simulink model "reaktor_nastawy"  (R2016a)
settings: Solver=VariableStepAuto  StartTime=0.0  StopTime=500  RelTol=1e-3
values from neighbouring files (symbols this model uses):
  B = 0.0064    [Unit_3.m]    (also in reactor_pocz.m; unit_1.m; unit_4.m)
  C_psi = 13.75 * (10 ^ 6)    (= 13750000)    [Unit_3.m]    (also in reactor_pocz.m; unit_4.m)
  LAMBDA = 10 ^ -5    (= 1e-05)    [Unit_3.m]    (also in reactor_pocz.m; unit_1.m; unit_4.m)
  lambda = 0.1    [Unit_3.m]    (also in reactor_pocz.m; unit_1.m; unit_4.m)
  P_1 = -1.223 * (10 ^ -4)    (= -0.0001223)    [Unit_3.m]    (also in reactor_pocz.m; unit_1.m = -0.0001322; unit_4.m = -0.0001286)
  P_2 = -5.502 * (10 ^ -5)    (= -5.502e-05)    [Unit_3.m]    (also in reactor_pocz.m; unit_1.m = -6.08e-05; unit_4.m = -6.79e-05)
  P_3 = -1.953 * (10 ^ -4)    (= -0.0001953)    [Unit_3.m]    (also in reactor_pocz.m; unit_1.m = -0.000285; unit_4.m = -0.0002887)
  S = 1938.9    [Unit_3.m]    (also in reactor_pocz.m; unit_1.m = 2859; unit_4.m = 2910.3)
libraries: simulink x2
settings Model: Creator=Użytkownik  LastModifiedBy=Użytkownik

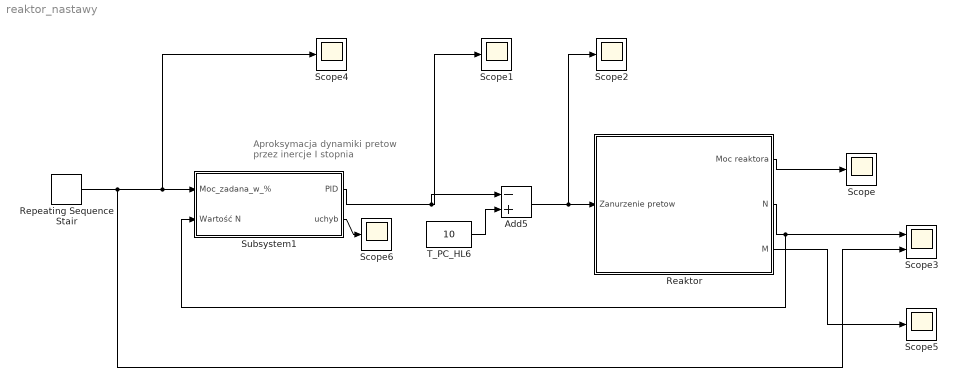
== system reaktor_nastawy ==
  note: Aproksymacja dynamiki
      | pretow przez inercje I stopnia
  Add5 : Sum  Inputs=-+
  Reaktor : Subsystem
  Repeating Sequence Stair : simulink/Sources/Repeating Sequence Stair  OutValues=[0 10 20 30 40 50 60 70 80 90 100].'  tsamp=50  OutMin=[]  OutMax=[]  OutDataTypeStr=double  OutputDataTypeScalingMode=double  OutDataType=fixdt(0,8)  ConRadixGroup=Best Precision: Vector-wise  OutScaling=2^-12
  Scope{,1..2,4..6} (6 alike) : Scope
  Scope3 : Scope  NumInputPorts=2
  Subsystem1 : Subsystem
  T_PC_HL6 : Constant  Value=10
  wires:
  Reaktor/1(Moc reaktora) -> Scope/1
  Repeating Sequence Stair/1 -> Scope3/2, Subsystem1/1(Moc_zadana_w_%), Scope4/1
  Subsystem1/1("PID ") -> Add5/1, Scope1/1
  Reaktor/2(N) -> Scope3/1, Subsystem1/2(Wartość N)
  Add5/1 -> Scope2/1, Reaktor/1(Zanurzenie pretow)
  T_PC_HL6/1 -> Add5/2
  Reaktor/3(M) -> Scope5/1
  Subsystem1/2(uchyb) -> Scope6/1

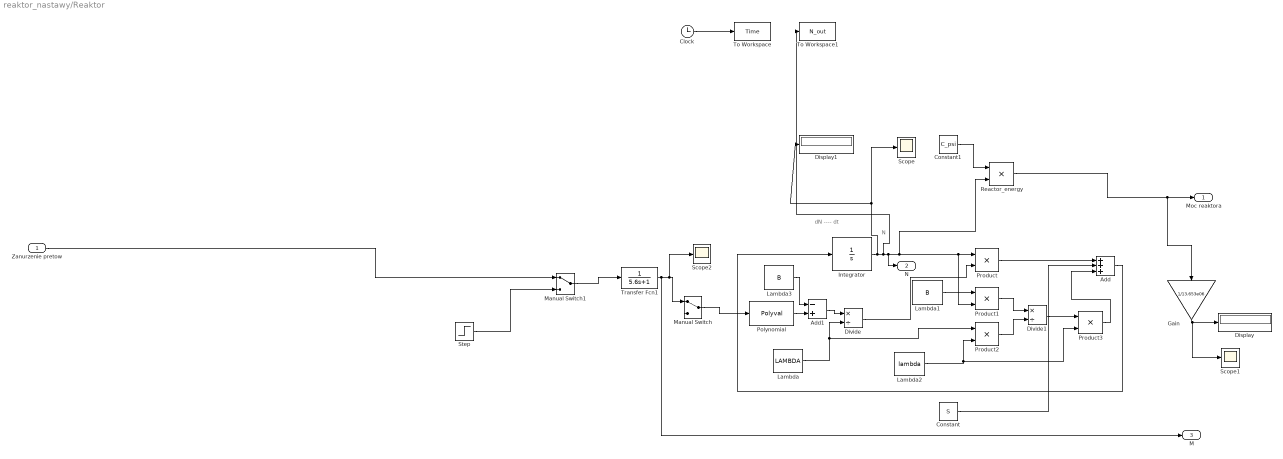
== system reaktor_nastawy/Reaktor ==
  note: N
  note: dN
      | ----
      | dt
  Zanurzenie pretow : Inport
  Add : Sum  Inputs=+++
  Add1 : Sum  Inputs=-+
  Clock : Clock
  Constant : Constant  Value=S
  Constant1 : Constant  Value=C_psi
  Display : Display
  Display1 : Display
  Divide : Product  Inputs=*/
  Divide1 : Product  Inputs=*/
  Gain : Gain  Gain=1/13.653e06
  Integrator : Integrator
  Lambda : Constant  Value=LAMBDA
  Lambda1 : Constant  Value=B
  Lambda2 : Constant  Value=lambda
  Lambda3 : Constant  Value=B
  Manual Switch : ManualSwitch
  Manual Switch1 : ManualSwitch
  Polynomial : Polyval  Coefs=[P_1, P_2, P_3]
  Product{,1..3} (4 alike) : Product
  Reactor_energy : Product
  Scope : Scope
  Scope1 : Scope
  Scope2 : Scope
  Step : Step  Time=10  Before=10  After=0.5449  SampleTime=0
  To Workspace : ToWorkspace  VariableName=Time  SampleTime=-1
  To Workspace1 : ToWorkspace  VariableName=N_out  SampleTime=-1
  Transfer Fcn1 : TransferFcn  Denominator=[5.6 1]
  Moc reaktora : Outport
  N : Outport  Port=2
  M : Outport  Port=3
  wires:
  Product/1 -> Add/1
  Constant/1 -> Add/2
  Add/1 -> Integrator/1
  Lambda/1 -> Product2/1, Divide/2
  Divide/1 -> Product/2
  Constant1/1 -> Reactor_energy/1
  Reactor_energy/1 -> Gain/1, Moc reaktora/1
  Lambda1/1 -> Product1/1
  Lambda2/1 -> Product2/2, Product3/2
  Product1/1 -> Divide1/1
  Product2/1 -> Divide1/2
  Divide1/1 -> Product3/1
  Product3/1 -> Add/3
  Lambda3/1 -> Add1/1
  Polynomial/1 -> Add1/2
  Add1/1 -> Divide/1
  Gain/1 -> Scope1/1, Display/1
  Transfer Fcn1/1 -> M/1, Scope2/1, Manual Switch/1
  Manual Switch/1 -> Polynomial/1
  Zanurzenie pretow/1 -> Manual Switch1/1
  Manual Switch1/1 -> Transfer Fcn1/1
  Step/1 -> Manual Switch1/2
  Integrator/1 -> To Workspace1/1, N/1, Reactor_energy/2, Product1/2, Product/1, Display1/1, Scope/1
  Clock/1 -> To Workspace/1

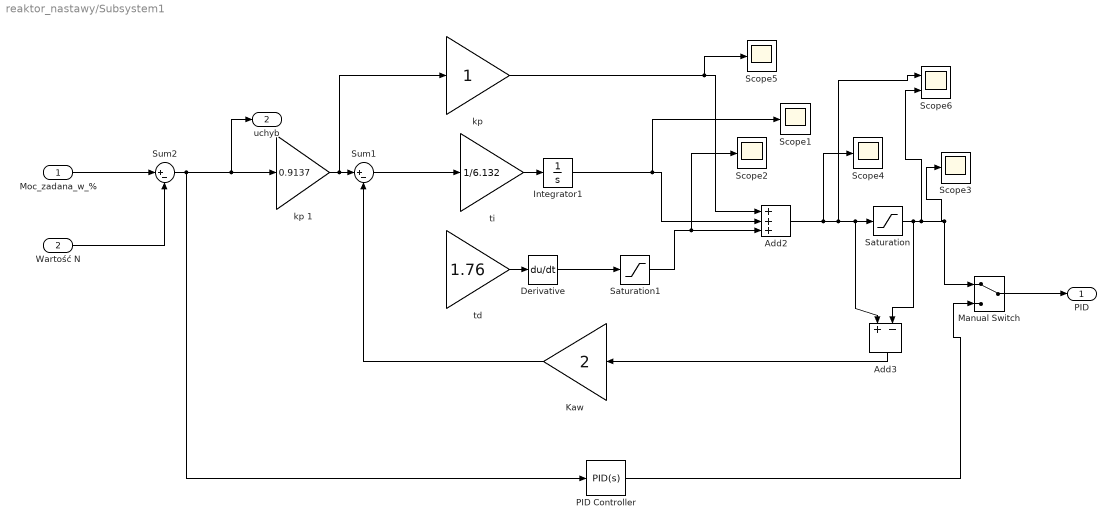
== system reaktor_nastawy/Subsystem1 ==
  Moc_zadana_w_% : Inport
  Wartość N : Inport  Port=2
  " kp " : Gain
  " kp 1" : Gain  Gain=0.9137
  Add2 : Sum  Inputs=+++
  Add3 : Sum  Inputs=+-
  Derivative : Derivative
  Integrator1 : Integrator
  "Kaw " : Gain  Gain=2
  Manual Switch : ManualSwitch
  PID Controller : simulink/Continuous/PID Controller  Controller=PID  TimeDomain=Continuous-time  SampleTime=-1  IntegratorMethod=Forward Euler  FilterMethod=Forward Euler  Form=Parallel  UseFilter=on  ControllerParametersSource=internal  P=0  I=-1  D=0  N=100  InitialConditionSource=internal  InitialConditionForIntegrator=0  InitialConditionForFilter=0  ExternalReset=none  LimitOutput=off  UpperSaturationLimit=inf  LowerSaturationLimit=-inf  LinearizeAsGain=on  AntiWindupMode=none  Kb=1  TrackingMode=off  Kt=1  PParamMin=[]  PParamMax=[]  IParamMin=[]  IParamMax=[]  DParamMin=[]  DParamMax=[]  NParamMin=[]  NParamMax=[]  KbParamMin=[]  KbParamMax=[]  KtParamMin=[]  KtParamMax=[]  POutMin=[]  POutMax=[]  IOutMin=[]  IOutMax=[]  DOutMin=[]  DOutMax=[]  NOutMin=[]  NOutMax=[]  KbOutMin=[]  KbOutMax=[]  KtOutMin=[]  KtOutMax=[]  IntegratorOutMin=[]  IntegratorOutMax=[]  FilterOutMin=[]  FilterOutMax=[]  SumOutMin=[]  SumOutMax=[]  SumI1OutMin=[]  SumI1OutMax=[]  SumI2OutMin=[]  SumI2OutMax=[]  SumI3OutMin=[]  SumI3OutMax=[]  SumDOutMin=[]  SumDOutMax=[]  SaturationOutMin=[]  SaturationOutMax=[]  IntegratorContinuousStateAttributes=''  IntegratorStateMustResolveToSignalObject=off  IntegratorRTWStateStorageClass=Auto  FilterContinuousStateAttributes=''  FilterStateMustResolveToSignalObject=off  FilterRTWStateStorageClass=Auto  DifferentiatorICPrevScaledInput=0  DifferentiatorOutMin=[]  DifferentiatorOutMax=[]
  Saturation : Saturate  UpperLimit=10  LowerLimit=0
  Saturation1 : Saturate  UpperLimit=10  LowerLimit=-10
  Scope{1..5} (5 alike) : Scope
  Scope6 : Scope  NumInputPorts=2
  Sum1 : Sum  Inputs=|+-
  Sum2 : Sum  Inputs=|+-
  "td " : Gain  Gain=1.76
  ti : Gain  Gain=1/6.132
  "PID " : Outport
  uchyb : Outport  Port=2
  wires:
  Derivative/1 -> Saturation1/1
  Add2/1 -> Scope6/1, Add3/1, Saturation/1, Scope4/1
  Saturation/1 -> Add3/2, Scope6/2, Scope3/1, Manual Switch/1
  Moc_zadana_w_%/1 -> Sum2/1
  Wartość N/1 -> Sum2/2
  Manual Switch/1 -> "PID "/1
  PID Controller/1 -> Manual Switch/2
  ti/1 -> Integrator1/1
  "td "/1 -> Derivative/1
  Add3/1 -> "Kaw "/1
  " kp 1"/1 -> " kp "/1, Sum1/1
  Sum1/1 -> ti/1
  Saturation1/1 -> Scope2/1, Add2/3
  Integrator1/1 -> Scope1/1, Add2/2
  " kp "/1 -> Scope5/1, Add2/1
  Sum2/1 -> uchyb/1, " kp 1"/1, PID Controller/1
  "Kaw "/1 -> Sum1/2
